simulink model "GPSIMUSignals"  (R2024b)
settings: configuration reference "STM32H7_Config" (kept outside this file)
settings Model: DataDictionary=Master_Dictionary.sldd  EnableAccessToBaseWorkspace=off  Creator=torni  LastModifiedBy=oxbro
settings ConfigSetRef: SourceName=STM32H7_Config

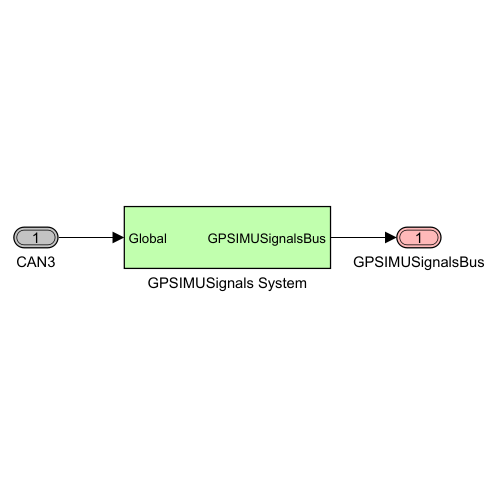
[thumbnail: Simulink's stored preview of the top-level diagram]
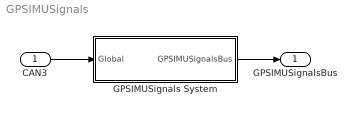
== system GPSIMUSignals ==
  CAN3 : Inport  OutDataTypeStr=Bus: CAN3Bus
  GPSIMUSignals System : Subsystem
  GPSIMUSignalsBus : Outport  OutDataTypeStr=Bus: GPSIMUSignalsBus  VectorParamsAs1DForOutWhenUnconnected=off
  wires:
  CAN3/1 -> GPSIMUSignals System/1(Global)
  GPSIMUSignals System/1(GPSIMUSignalsBus) -> GPSIMUSignalsBus/1

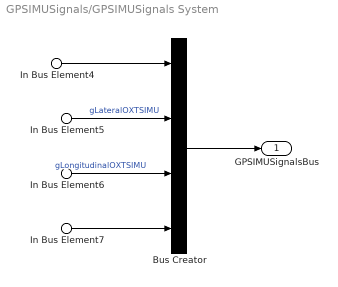
== system GPSIMUSignals/GPSIMUSignals System ==
  In Bus Element4 : Inport  PortName=Global  Element=OXTSDataFrame1540.vLongitudinalOXTSIMU
  In Bus Element5 : Inport  PortName=Global  Element=OXTSDataFrame1541.gLateralOXTS
  In Bus Element6 : Inport  PortName=Global  Element=OXTSDataFrame1541.gLongitudinalOXTS
  In Bus Element7 : Inport  PortName=Global  Element=OXTSDataFrame1544.nYawRateOXTSIMU
  Bus Creator : BusCreator  Inputs=4  OutDataTypeStr=Bus: GPSIMUSignalsBus
  GPSIMUSignalsBus : Outport  OutDataTypeStr=Bus: GPSIMUSignalsBus  VectorParamsAs1DForOutWhenUnconnected=off
  wires:
  Bus Creator/1 -> GPSIMUSignalsBus/1
  In Bus Element4/1 -> Bus Creator/1
  In Bus Element5/1 -> Bus Creator/2  "gLateralOXTSIMU"
  In Bus Element6/1 -> Bus Creator/3  "gLongitudinalOXTSIMU"
  In Bus Element7/1 -> Bus Creator/4
